simulink model "Main_bikesim"  (R2022b)
settings: Solver=FixedStepAuto  StartTime=0.0  StopTime=sim_time-0.02  FixedStep=0.005
values from neighbouring files (symbols this model uses):
  A_d = (eye(size(A))+Ts*A)    [Kalman_offline.m]    (also in Main_sim.m; Startup_labview.m)
  Ad_t = (eye(size(A_t))+Ts*A_t)    [Main_sim.m]    (also in Startup_labview.m)
  B_d = Ts*B    [Kalman_offline.m]    (also in Main_sim.m; Startup_labview.m)
  Bd_t = B_t*Ts    [Main_sim.m]    (also in Startup_labview.m)
  bike_model = 1    [Main_sim.m]
  bike_params = LoadBikeParameters(bike)    [Kalman_offline.m]    (also in Main_sim.m; Startup_labview.m)
  C1 = [1 0 0 0 0 0 0 ... (first row only)    [Kalman_offline.m]    (also in Main_sim.m; Startup_labview.m)
  C2 = [(-g+((-h_imu*g)/h)) 0 (-h_imu*(h*v^2-(g*lr*c)))*sin(lambda)/((lr+lf)*h^2)+(v^2)*sin(lambda)/(lr+lf) 0 ... (first row only)    [Kalman_offline.m]    (also in Main_sim.m; Startup_labview.m)
  counter = (Ts_GPS / Ts) - 1    (= 9)    [Kalman_offline.m]    (also in Main_sim.m; Startup_labview.m)
  D1 = [0 0 (-h_imu*lr*v)/((lr+lf)*h) 0 0 0 0]'    [Kalman_offline.m]    (also in Main_sim.m; Startup_labview.m)
  D2 = [(-h_imu*lr*v)/((lr+lf)*h) 0 0 0 0]'    [Kalman_offline.m]    (also in Main_sim.m; Startup_labview.m)
  e1_max = abs(-k2*e2_max/k1)    [Main_sim.m]    (also in Startup_labview.m)
  g = 9.81    [Kalman_offline.m]    (also in Main_sim.m; Startup_labview.m)
  hor_dis = 10    [Main_sim.m]
  I_balancing_outer = 0.0    (= 0)    [Main_sim.m]    (also in Startup_labview.m)
  initial_state_estimate = initial_state    [Kalman_offline.m]    (also in Main_sim.m)
  k1 = K(1)    [Main_sim.m]    (also in Startup_labview.m)
  k2 = K(2)    [Main_sim.m]    (also in Startup_labview.m)
  Kalman_gain1 = Kalman_gain1'    [Kalman_offline.m]    (also in Main_sim.m; Startup_labview.m)
  Kalman_gain2 = Kalman_gain1(4:7,3:7)    [Kalman_offline.m]    (also in Main_sim.m; Startup_labview.m)
  P_balancing_inner = 3    [Main_sim.m]    (also in Startup_labview.m = 1)
  P_balancing_outer = 1.3    [Main_sim.m]    (also in Startup_labview.m = 1.75)
  ref_dis = 0.01    [Main_sim.m]
  ref_start_idx = 2    [Main_sim.m]
  T = Rz*Ry*Rx    [Kalman_offline.m]    (also in Main_sim.m)
  Ts = 0.01    [Kalman_offline.m]    (also in Main_sim.m; Startup_labview.m)
  v = 2    [Kalman_offline.m]    (also in Main_sim.m; Startup_labview.m)
undefined symbols (not defined in the file or in its folder): C_t, D_t, initial_state, linearized_sys, pert_deltadot_state, pert_deltadot_state_fun, pert_phidot_state, pert_phidot_state_fun, Psiref, sigbuilder_block, Xref, Yref
libraries: simulink x8, slpidlib x2, eeGeneralControl x1
(part 2 of 2)

== matlab function Main_bikesim/Trajectory controller1/Trajectory controller ==
  settings: updateMethod=DISCRETE  sampleTime=Ts
  data: e1 output; e2 output; closestpoint_idx output; closestpoint_heading_idx output; Xref_loc input; Yref_loc input; psiref_loc input; X_est input; Y_est input; psi_est input; bike_params input; traj_error_params input; ref_X output; ref_Y output; ref_psi output; v input; roll_ref output; delta_ref output; x input; x_dot output; Ad_t parameter; Bd_t parameter; C_t parameter; D_t parameter
function [e1,e2,closestpoint_idx,closestpoint_heading_idx,ref_X,ref_Y,ref_psi,roll_ref,delta_ref,x_dot]= fcn(Xref_loc,Yref_loc,psiref_loc,X_est,Y_est,psi_est,bike_params,traj_error_params, ...
                                                                                                            v, x, Ad_t, Bd_t, C_t, D_t)
%% calculations on a local part of the trajectory

% Unpack parameters
g  = bike_params(1);
lr = bike_params(2);
lf = bike_params(3);
lambda = bike_params(4);

k1 = traj_error_params(1);
k2 = traj_error_params(2);
e1_max = traj_error_params(3);

% Each referencepoint has a location (X,Y) and a heading
% The heading is defined in the startup.m file as 'the heading where its coming from' 
% Second point in local reference is current selected closest point
closestpoint_idx=2;

% Search for closest point
% Finding the closest point going forward. Stop searching once next
% distance increases

while (Xref_loc(closestpoint_idx,1)-X_est)^2 + (Yref_loc(closestpoint_idx,1)-Y_est)^2 >= (Xref_loc(closestpoint_idx+1,1)-X_est)^2+(Yref_loc(closestpoint_idx+1,1)-Y_est)^2  && closestpoint_idx <= length(Xref_loc)-2
closestpoint_idx = closestpoint_idx+1;
end

% Select same closest point (for heading error and position error)
closestpoint_heading_idx = closestpoint_idx;


% Calculate X and Y distance from current location to selected closest
% point
dx = X_est - Xref_loc(closestpoint_idx,1);
dy = Y_est - Yref_loc(closestpoint_idx,1);

% Calculate difference in current heading and heading in reference point 
% And limit D_psiref  between -2pi and 2pi
D_psiref=psiref_loc(closestpoint_idx+1,1)-psiref_loc(closestpoint_idx,1);
if D_psiref>=pi
    D_psiref=mod(D_psiref,-2*pi);
end
if D_psiref<=-pi
    D_psiref=mod(D_psiref,2*pi);
end
%IMPROVEMENT: implement an interpolation algoritm
% Calculate distence between point before closest point and current location
dist_true_previous = sqrt((Xref_loc(closestpoint_idx-1,1)-X_est)^2+(Yref_loc(closestpoint_idx-1,1)-Y_est)^2);
% Angle of line between previous closest point and current location
alpha_star = atan((Yref_loc(closestpoint_idx-1,1)-Y_est)/(Xref_loc(closestpoint_idx-1,1)-X_est));
% heading previous closest point - alpha star
alpha_projected_dist = alpha_star-psiref_loc(closestpoint_idx,1);
% the distance from the previous closest point to the projection of the bike on the trajectory
Projected_dist = abs(dist_true_previous*cos(alpha_projected_dist));

compared_dist = sqrt((Xref_loc(closestpoint_idx,1)-Xref_loc(closestpoint_idx-1,1))^2+(Yref_loc(closestpoint_idx,1)-Yref_loc(closestpoint_idx-1,1))^2);

% If bike passes closest point, the heading of the next point will be taken
if Projected_dist >= compared_dist
closestpoint_heading_idx = closestpoint_idx+1;
end

%calculate e1 and e2        
e1= dy*cos(psiref_loc(closestpoint_heading_idx,1)) - dx*sin(psiref_loc(closestpoint_heading_idx,1)); % this make e1 include "direction" automatically
e2= psi_est-psiref_loc(closestpoint_heading_idx,1); %calculate e2

% closest point on the local trajectory
ref_X=Xref_loc(closestpoint_idx,1);
ref_Y=Yref_loc(closestpoint_idx,1);
ref_psi=psiref_loc(closestpoint_heading_idx,1);

 % keep heading error should be between -pi 2 pi
e2 = wrapToPi(e2);
%e2=mod(e2+pi,2*pi)-pi;     

%calculate the time between psiref(idx,1) and psiref(idx+1,1)
dX=Xref_loc(closestpoint_idx+1,1)-ref_X;
dY=Yref_loc(closestpoint_idx+1,1)-ref_Y;
dis=sqrt(dX^2+dY^2);
Ts_psi=dis/v;

% Sample dpsiref
dpsiref=(D_psiref)/Ts_psi;

% Reset closest point index as feedback for local frame selection
closestpoint_idx = closestpoint_idx-1;

% Steering contribution from trajectory error
delta_ref_error=-k1*sign(e1)*min(abs(e1),e1_max)-k2*e2;

% Steering contribution from heading change
x_dot = Ad_t*x + Bd_t*dpsiref;
delta_ref_psi = C_t*x + D_t*dpsiref; 

% Total steering reference 
delta_ref = delta_ref_psi + delta_ref_error;

% limit steer angle between -pi/4 and pi/4
if delta_ref>=pi/4
    delta_ref=pi/4;
end

if delta_ref<=-pi/4
    delta_ref=-pi/4;
end

% Transform steering reference into roll reference for balancing controller
eff_delta_ref = delta_ref*sin(lambda);
roll_ref = -1*atan((tan(eff_delta_ref)*(v^2/(lr+lf)))/g);








end

== matlab function Main_bikesim/Selection of local reference from total reference1/Local reference selection & stop funcion ==
  data: last_ids input; ids output; xref input; local_Xref output size=Nn [..30000]; local_Yref output size=Nn [..30000]; local_Psiref output size=Nn [..30000]; yref input; psiref input; closest_point input; ref_dis parameter; hor_dis parameter; stop output
function [ids,local_Xref,local_Yref,local_Psiref,stop] = fcn(last_ids,xref,yref,psiref,closest_point, ref_dis, hor_dis)
% Local reference trajectory starts at point before the current closest
% point and has a length of M
ids=last_ids+closest_point-1;      % calculate the initial index of the points that will be sent to next block (first point of local_ref)

Ns=ceil(hor_dis/ref_dis);          % Th,Ts is definited in "StudentProject2021.m", Ns is the number of points sent to next block
M=ids+Ns;                          % calculate the end index of the end index that will be sent to next block
n=size(xref,1);                    % size of whole trajectory points 
if M>n                             % if reached near end of reference, local trajectry becomes shorter
    M=n;
end

% Temporary simulation STOP to prevent singularity error once approaching
% the end of the trajectory
% Simulation stops before the end of the reference trajectory
stop = 0;
if ids>=n-ceil(n/10)
    stop = 1;
end

% Start always at second value of total reference
% if ids == 1
% ids = 2;
% end

% Select local reference from total reference
local_Xref=xref(ids-1:M,1);
local_Yref=yref(ids-1:M,1);
local_Psiref=psiref(ids-1:M,1);

== matlab function Main_bikesim/Subsystem/Trajectory controller ==
  settings: updateMethod=DISCRETE  sampleTime=Ts
  data: closestpoint_idx_in input; closestpoint_idx_out output; e1 output; e2 output; closestpoint_heading_idx output; Xref_loc input; Yref_loc input; psiref_loc input; X_est input; Y_est input; psi_est input; bike_params input; traj_error_params input; ref_X output; ref_Y output; ref_psi output; v input; roll_ref output; delta_ref output; x input; x_dot output; Ad_t parameter; Bd_t parameter; C_t parameter; D_t parameter; delta_e1 output; delta_e2 output
function [closestpoint_idx_out,e1,e2,closestpoint_heading_idx,ref_X,ref_Y,ref_psi,roll_ref,delta_ref,x_dot,delta_e1,delta_e2]= fcn(closestpoint_idx_in,Xref_loc,Yref_loc,psiref_loc,X_est,Y_est,psi_est,bike_params,traj_error_params, ...
                                                                                                            v, x, Ad_t, Bd_t, C_t, D_t)
%% calculations on a local part of the trajectory

% Unpack parameters
g  = bike_params(1);
lr = bike_params(2);
lf = bike_params(3);
lambda = bike_params(4);

k1 = traj_error_params(1);
k2 = traj_error_params(2);
e1_max = traj_error_params(3);

% Search for closest point
% Finding the closest point going forward. Stop searching once next
% distance increases

while (Xref_loc(closestpoint_idx_in,1)-X_est)^2 + (Yref_loc(closestpoint_idx_in,1)-Y_est)^2 >= (Xref_loc(closestpoint_idx_in+1,1)-X_est)^2+(Yref_loc(closestpoint_idx_in+1,1)-Y_est)^2  && closestpoint_idx_in <= length(Xref_loc)-2
closestpoint_idx_in = closestpoint_idx_in+1;
end

% Select same closest point (for heading error and position error)
closestpoint_heading_idx = closestpoint_idx_in;


% Calculate X and Y distance from current location to selected closest
% point
dx = X_est - Xref_loc(closestpoint_idx_in,1);
dy = Y_est - Yref_loc(closestpoint_idx_in,1);

% Calculate difference in current heading and heading in reference point 
% And limit D_psiref  between -2pi and 2pi
D_psiref=psiref_loc(closestpoint_idx_in+1,1)-psiref_loc(closestpoint_idx_in,1);
if D_psiref>=pi
    D_psiref=mod(D_psiref,-2*pi);
end
if D_psiref<=-pi
    D_psiref=mod(D_psiref,2*pi);
end
%IMPROVEMENT: implement an interpolation algoritm
% Calculate distence between point before closest point and current location
dist_true_previous = sqrt((Xref_loc(closestpoint_idx_in-1,1)-X_est)^2+(Yref_loc(closestpoint_idx_in-1,1)-Y_est)^2);
% Angle of line between previous closest point and current location
alpha_star = atan((Yref_loc(closestpoint_idx_in-1,1)-Y_est)/(Xref_loc(closestpoint_idx_in-1,1)-X_est));
% heading previous closest point - alpha star
alpha_projected_dist = alpha_star-psiref_loc(closestpoint_idx_in,1);
% the distance from the previous closest point to the projection of the bike on the trajectory
Projected_dist = abs(dist_true_previous*cos(alpha_projected_dist));

compared_dist = sqrt((Xref_loc(closestpoint_idx_in,1)-Xref_loc(closestpoint_idx_in-1,1))^2+(Yref_loc(closestpoint_idx_in,1)-Yref_loc(closestpoint_idx_in-1,1))^2);

% If bike passes closest point, the heading of the next point will be taken
if Projected_dist >= compared_dist
closestpoint_heading_idx = closestpoint_idx_in+1;
end

%calculate e1 and e2        
e1= dy*cos(psiref_loc(closestpoint_heading_idx,1)) - dx*sin(psiref_loc(closestpoint_heading_idx,1)); % this make e1 include "direction" automatically
e2= psi_est-psiref_loc(closestpoint_heading_idx,1); %calculate e2

% closest point on the local trajectory
ref_X=Xref_loc(closestpoint_idx_in,1);
ref_Y=Yref_loc(closestpoint_idx_in,1);
ref_psi=psiref_loc(closestpoint_heading_idx,1);

 % keep heading error should be between -pi 2 pi
e2 = wrapToPi(e2);
%e2=mod(e2+pi,2*pi)-pi;     

%calculate the time between psiref(idx,1) and psiref(idx+1,1)
dX=Xref_loc(closestpoint_idx_in+1,1)-ref_X;
dY=Yref_loc(closestpoint_idx_in+1,1)-ref_Y;
dis=sqrt(dX^2+dY^2);
Ts_psi=dis/v;

% Sample dpsiref
dpsiref=(D_psiref)/Ts_psi;

% Loop the closest point
closestpoint_idx_out = closestpoint_idx_in;

% Steering contribution from trajectory error
delta_ref_error=-k1*sign(e1)*min(abs(e1),e1_max)-k2*e2;
delta_e1 = -k1*sign(e1)*min(abs(e1),e1_max);
delta_e2 =-k2*e2;

% Steering contribution from heading change
x_dot = Ad_t*x + Bd_t*dpsiref;
delta_ref_psi = C_t*x + D_t*dpsiref; 

% Total steering reference 
delta_ref = delta_ref_psi + delta_ref_error;

% limit steer angle between -pi/4 and pi/4
if delta_ref>=pi/4
    delta_ref=pi/4;
end

if delta_ref<=-pi/4
    delta_ref=-pi/4;
end

% Transform steering reference into roll reference for balancing controller
eff_delta_ref = delta_ref*sin(lambda);
roll_ref = -1*atan(tan(eff_delta_ref)*(v^2/(lr+lf))/g);








end

== matlab function Main_bikesim/Sensors1/Define true sensor positions on the bike ==
  data: bike_params input; pose input; pose_corrected output
function pose_corrected  = fcn(bike_params, pose)
pose_corrected = pose;

gpsX = bike_params(1); % measured offset of GPS parallel to bike
gpsY = bike_params(2); % measured offset of GPS perpendicular to bike
gpsH = bike_params(3); % measured offset of GPS from ground to GPS

% define pose_l
pose_l = pose;

% Transform to local frame
    pose_l(1) =  pose(1) * cos(pose(3)) + pose(2) * sin(pose(3));
    pose_l(2) = -pose(1) * sin(pose(3)) + pose(2) * cos(pose(3)); 

% define actual positions of GPS 
% pose1 = difference in x in local frame
% pose2 = difference in y in local frame
    pose_l(1) = pose_l(1) + gpsX;
    pose_l(2) = pose_l(2) + gpsY + gpsH*sin(pose(4));

% define actual positions of IMU 


% Transform back to global frame
    pose(1) = pose_l(1) * cos(pose(3)) - pose_l(2) * sin(pose(3));
    pose(2) = pose_l(1) * sin(pose(3)) + pose_l(2) * cos(pose(3));

pose_corrected(1) = pose(1);
pose_corrected(2) = pose(2);
